simulink model "basic_FC"  (R2023b)
settings: Solver=VariableStepAuto  StartTime=0.0  StopTime=3600*8760*3  MaxStep=1000  RelTol=1e-5
values from neighbouring files (symbols this model uses):
  I_s_0 = 1.85    [fuelCycleSimulator.m]    (also in parametric_analysis_f_p_trap.m = 0.8; utilities.m = I_s_0 - abs(margin) + inventory_accuracy)
  N_dot = 9.3e-7    (= 9.3e-07)    [FC_scenario_inputData.m]    (also in inputData.m)
  n_trap = n_trap_array(j)    [parametric_analysis_trapping.m]
  TBR = 1.096    [fuelCycleSimulator.m]    (also in parametric_analysis_f_p_trap.m = 1.048; parametric_analysis_trapping.m = 1.06; utilities.m = TBR_start)
undefined symbols (not defined in the file or in its folder): arc, f_b, fuelCleanUp_8, storage_10, tau_detrap, tau_ifc, tau_ofc
settings Model: Creator=smesc  LastModifiedBy=smesc
settings SolverCC: InitialStep=1e-4
settings ModelReferenceCC: EnableRefExpFcnMdlSchedulingChecks=on

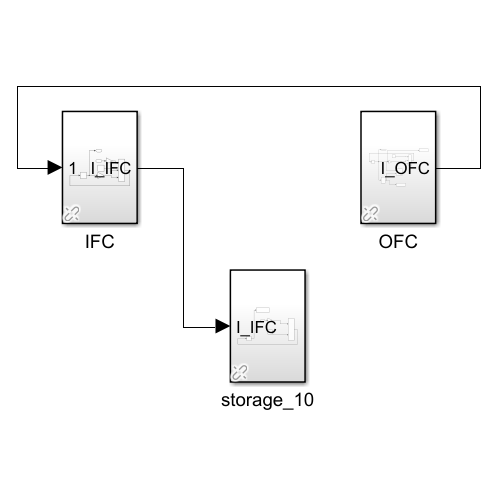
[thumbnail: Simulink's stored preview of the top-level diagram]
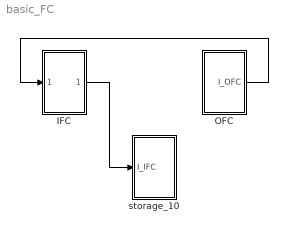
== system basic_FC ==
  IFC : Subsystem  AncestorBlock=arc/fuelCleanUp_8
  OFC : Subsystem  AncestorBlock=arc/fuelCleanUp_8
  storage_10 : Subsystem  AncestorBlock=arc/storage_10
  wires:
  OFC/1(I_OFC) -> IFC/1(Input)
  IFC/1(I_IFC) -> storage_10/1(I_IFC)

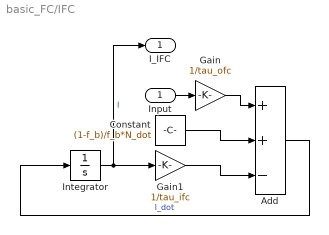
== system basic_FC/IFC ==
  Input : Inport
  Add : Sum  Inputs=++-
  Constant : Constant  Value=(1-f_b)/f_b*N_dot
  Gain : Gain  Gain=1/tau_ofc
  Gain1 : Gain  Gain=1/tau_ifc
  Integrator : Integrator
  I_IFC : Outport
  wires:
  Input/1 -> Gain/1
  Add/1 -> Integrator/1  "I_dot"
  Integrator/1 -> Gain1/1, I_IFC/1  "I"
  Gain/1 -> Add/1
  Gain1/1 -> Add/3
  Constant/1 -> Add/2

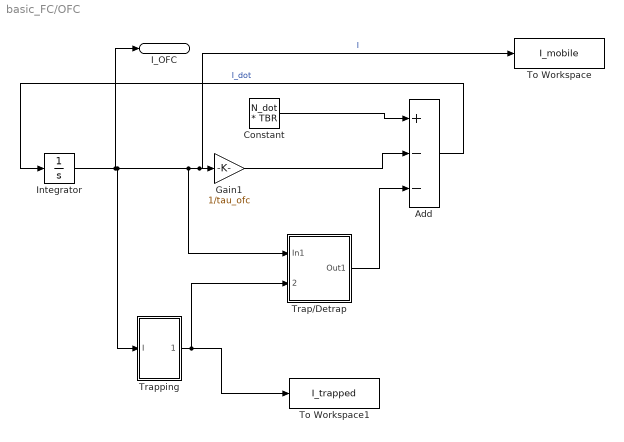
== system basic_FC/OFC ==
  Add : Sum  Inputs=+--
  Constant : Constant  Value=N_dot * TBR
  Gain1 : Gain  Gain=1/tau_ofc
  Integrator : Integrator
  To Workspace : ToWorkspace  VariableName=I_mobile  SampleTime=-1
  To Workspace1 : ToWorkspace  VariableName=I_trapped  SampleTime=-1
  Trap/Detrap : Subsystem
  Trapping : Subsystem
  I_OFC : Outport
  wires:
  Gain1/1 -> Add/2
  Add/1 -> Integrator/1  "I_dot"
  Integrator/1 -> Trap/Detrap/1(In1), To Workspace/1, Gain1/1, Trapping/1(I), I_OFC/1  "I"
  Constant/1 -> Add/1
  Trapping/1(Output) -> Trap/Detrap/2(Output), To Workspace1/1
  Trap/Detrap/1(Out1) -> Add/3

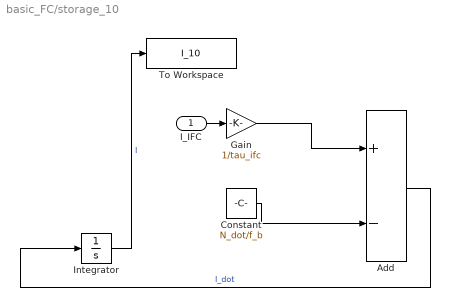
== system basic_FC/storage_10 ==
  I_IFC : Inport
  Add : Sum  Inputs=+-
  Constant : Constant  Value=N_dot/f_b
  Gain : Gain  Gain=1/tau_ifc
  Integrator : Integrator  InitialCondition=I_s_0
  To Workspace : ToWorkspace  VariableName=I_10  SampleTime=-1
  wires:
  Integrator/1 -> To Workspace/1  "I"
  Add/1 -> Integrator/1  "I_dot"
  Constant/1 -> Add/2
  I_IFC/1 -> Gain/1
  Gain/1 -> Add/1

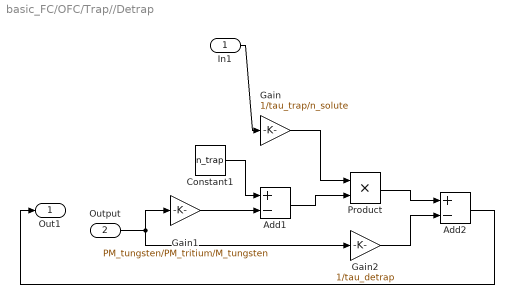
== system basic_FC/OFC/Trap//Detrap ==
  In1 : Inport
  Output : Inport  Port=2
  Add1 : Sum  Inputs=+-
  Add2 : Sum  Inputs=+-
  Constant1 : Constant  Value=n_trap
  Gain : Gain  Gain=1/tau_trap/n_solute
  Gain1 : Gain  Gain=PM_tungsten/PM_tritium/M_tungsten
  Gain2 : Gain  Gain=1/tau_detrap
  Product : Product
  Out1 : Outport
  wires:
  Product/1 -> Add2/1
  Add2/1 -> Out1/1
  In1/1 -> Gain/1
  Gain/1 -> Product/1
  Constant1/1 -> Add1/1
  Gain2/1 -> Add2/2
  Add1/1 -> Product/2
  Gain1/1 -> Add1/2
  Output/1 -> Gain2/1, Gain1/1

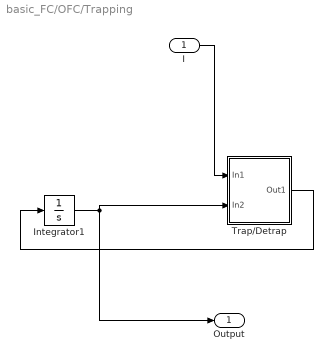
== system basic_FC/OFC/Trapping ==
  I : Inport
  Integrator1 : Integrator
  Trap/Detrap : Subsystem
  Output : Outport
  wires:
  Integrator1/1 -> Output/1, Trap/Detrap/2(In2)
  I/1 -> Trap/Detrap/1(In1)
  Trap/Detrap/1(Out1) -> Integrator1/1

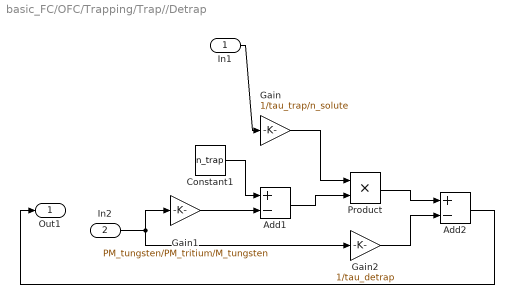
== system basic_FC/OFC/Trapping/Trap//Detrap ==
  In1 : Inport
  In2 : Inport  Port=2
  Add1 : Sum  Inputs=+-
  Add2 : Sum  Inputs=+-
  Constant1 : Constant  Value=n_trap
  Gain : Gain  Gain=1/tau_trap/n_solute
  Gain1 : Gain  Gain=PM_tungsten/PM_tritium/M_tungsten
  Gain2 : Gain  Gain=1/tau_detrap
  Product : Product
  Out1 : Outport
  wires:
  Product/1 -> Add2/1
  Add2/1 -> Out1/1
  In1/1 -> Gain/1
  Gain/1 -> Product/1
  Constant1/1 -> Add1/1
  Gain2/1 -> Add2/2
  Add1/1 -> Product/2
  Gain1/1 -> Add1/2
  In2/1 -> Gain2/1, Gain1/1
